simulink model "FA_18_With_Controller_Multiple_Actuator_Failure"  (R2018a)
settings: Solver=ode45  StartTime=0.0  StopTime=50  RelTol=1e-3
PreLoadFcn:
  | F18_Linear
values from neighbouring files (symbols this model uses):
  C1 = [0 -1 0 1]    [F18_Linear.m]
  d2r = pi/180    (= 0.0174532925199)    [F18_Linear.m]    (also in FA_18_Trim.m; FA_18_sfun.m; Sim.m)
  F1 = [-67.81 11973 -133.3 -11801]    [F18_Linear.m]
  F2 = 1414.2    [F18_Linear.m]
  Trimx_N = [365.74;15*d2r;0;15*d2r]    [F18_Linear.m]
undefined symbols (not defined in the file or in its folder): Earth, WGS84
libraries: aerolibfltsims x1, aerolibtransform2 x1, aerolibconvert2 x1
settings Model: Creator=User  LastModifiedBy=User

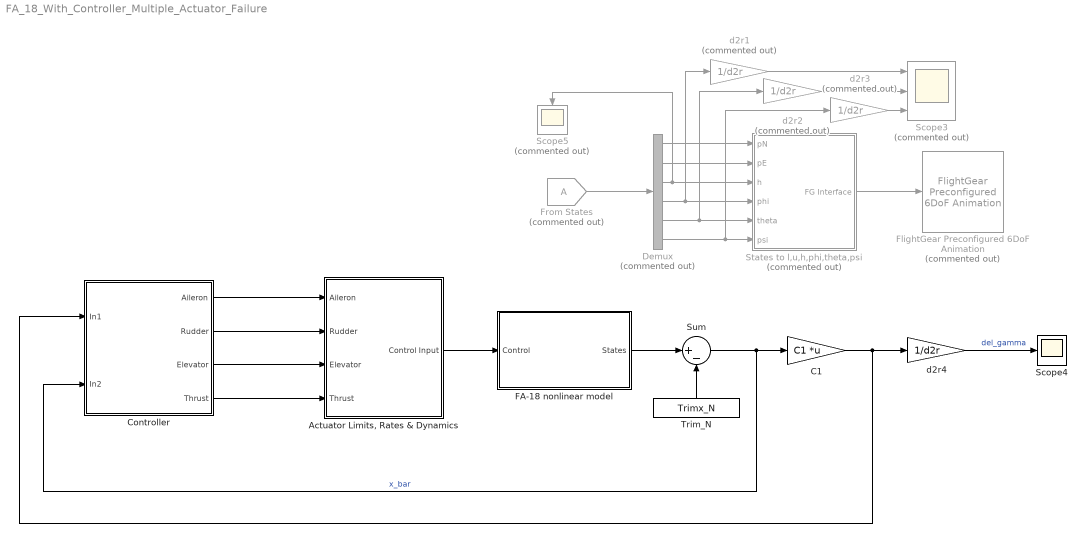
== system FA_18_With_Controller_Multiple_Actuator_Failure ==
  "Actuator Limits, Rates & Dynamics" : Subsystem
  C1 : Gain  Gain=C1  Multiplication=Matrix(K*u)
  Controller : Subsystem
  Demux : Demux  Commented=on  Outputs=6
  FA-18 nonlinear model : Subsystem
  FlightGear Preconfigured 6DoF Animation : aerolibfltsims/FlightGear Preconfigured 6DoF Animation  Commented=on  xFlightGearVersion=v2017.3  DestinationIpAddress=127.0.0.1  DestinationPort=5502  SampleTime=1/30
      settings: SourceProductName=Aerospace Blockset
  From States : From  Commented=on  TagVisibility=global
  Scope3 : Scope  Commented=on  NumInputPorts=3
  Scope4 : Scope
  Scope5 : Scope  Commented=on
  States to l,u,h,phi,theta,psi : Subsystem  Commented=on
  Sum : Sum  Inputs=|+-
  Trim_N : Constant  Value=Trimx_N
  d2r1 : Gain  Commented=on  Gain=1/d2r
  d2r2 : Gain  Commented=on  Gain=1/d2r
  d2r3 : Gain  Commented=on  Gain=1/d2r
  d2r4 : Gain  Gain=1/d2r
  wires:
  "Actuator Limits, Rates & Dynamics"/1(Control Input) -> FA-18 nonlinear model/1(Control)
  FA-18 nonlinear model/1(States) -> Sum/1
  Trim_N/1 -> Sum/2
  d2r4/1 -> Scope4/1  "del_gamma"
  C1/1 -> Controller/1(In1), d2r4/1
  Sum/1 -> Controller/2(In2), C1/1  "x_bar"
  States to l,u,h,phi,theta,psi/1(FG Interface) -> FlightGear Preconfigured 6DoF Animation/1
  From States/1 -> Demux/1
  Demux/1 -> States to l,u,h,phi,theta,psi/1(pN)
  Demux/2 -> States to l,u,h,phi,theta,psi/2(pE)
  Demux/5 -> States to l,u,h,phi,theta,psi/5(theta), d2r2/1
  Demux/6 -> d2r3/1, States to l,u,h,phi,theta,psi/6(psi)
  Demux/4 -> d2r1/1, States to l,u,h,phi,theta,psi/4(phi)
  d2r1/1 -> Scope3/1
  d2r2/1 -> Scope3/2
  d2r3/1 -> Scope3/3
  Demux/3 -> Scope5/1, States to l,u,h,phi,theta,psi/3(h)
  Controller/1(Aileron) -> "Actuator Limits, Rates & Dynamics"/1(Aileron)
  Controller/2(Rudder) -> "Actuator Limits, Rates & Dynamics"/2(Rudder)
  Controller/3("Elevator ") -> "Actuator Limits, Rates & Dynamics"/3(Elevator)
  Controller/4(Thrust) -> "Actuator Limits, Rates & Dynamics"/4(Thrust)

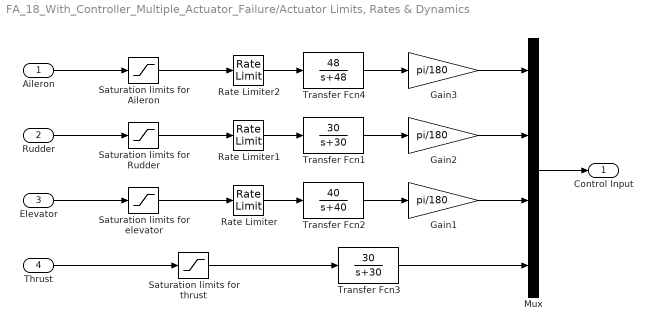
== system FA_18_With_Controller_Multiple_Actuator_Failure/Actuator Limits, Rates & Dynamics ==
  Aileron : Inport
  Rudder : Inport  Port=2
  Elevator : Inport  Port=3
  Thrust : Inport  Port=4
  Gain1 : Gain  Gain=pi/180
  Gain2 : Gain  Gain=pi/180
  Gain3 : Gain  Gain=pi/180
  Mux : Mux
  Rate Limiter : RateLimiter  RisingSlewLimit=40  FallingSlewLimit=-40  SampleTimeMode=inherited
  Rate Limiter1 : RateLimiter  RisingSlewLimit=61  FallingSlewLimit=-61  SampleTimeMode=inherited
  Rate Limiter2 : RateLimiter  RisingSlewLimit=100  FallingSlewLimit=-100  SampleTimeMode=inherited
  Saturation limits for Aileron : Saturate  UpperLimit=45  LowerLimit=-25
  Saturation limits for Rudder : Saturate  UpperLimit=30  LowerLimit=30
  Saturation limits for elevator : Saturate  UpperLimit=10.5  LowerLimit=-24
  Saturation limits for thrust : Saturate  UpperLimit=20000  LowerLimit=0
  Transfer Fcn1 : TransferFcn  Numerator=[30]  Denominator=[1 30]
  Transfer Fcn2 : TransferFcn  Numerator=[40]  Denominator=[1 40]
  Transfer Fcn3 : TransferFcn  Numerator=[30]  Denominator=[1 30]
  Transfer Fcn4 : TransferFcn  Numerator=[48]  Denominator=[1 48]
  Control Input : Outport
  wires:
  Mux/1 -> Control Input/1
  Thrust/1 -> Saturation limits for thrust/1
  Transfer Fcn3/1 -> Mux/4
  Saturation limits for thrust/1 -> Transfer Fcn3/1
  Saturation limits for elevator/1 -> Rate Limiter/1
  Rate Limiter/1 -> Transfer Fcn2/1
  Elevator/1 -> Saturation limits for elevator/1
  Gain1/1 -> Mux/3
  Transfer Fcn2/1 -> Gain1/1
  Saturation limits for Aileron/1 -> Rate Limiter2/1
  Aileron/1 -> Saturation limits for Aileron/1
  Rudder/1 -> Saturation limits for Rudder/1
  Saturation limits for Rudder/1 -> Rate Limiter1/1
  Rate Limiter1/1 -> Transfer Fcn1/1
  Rate Limiter2/1 -> Transfer Fcn4/1
  Transfer Fcn4/1 -> Gain3/1
  Transfer Fcn1/1 -> Gain2/1
  Gain2/1 -> Mux/2
  Gain3/1 -> Mux/1

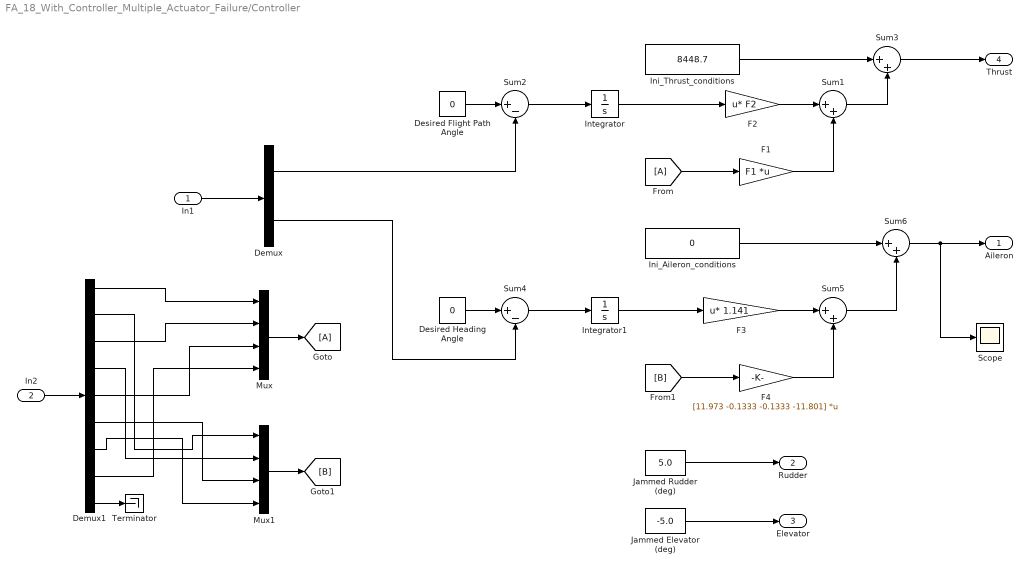
== system FA_18_With_Controller_Multiple_Actuator_Failure/Controller ==
  In1 : Inport
  In2 : Inport  Port=2
  Demux : Demux  Outputs=2
  Demux1 : Demux  Outputs=9
  Desired Flight Path Angle : Constant  Value=0
  Desired Heading Angle : Constant  Value=0
  F1 : Gain  Gain=F1  Multiplication=Matrix(K*u)
  F2 : Gain  Gain=F2  Multiplication=Matrix(u*K)
  F3 : Gain  Gain=1.141  Multiplication=Matrix(u*K)
  F4 : Gain  Gain=[11.973 -0.1333 -0.1333 -11.801]  Multiplication=Matrix(K*u)
  Ini_Aileron_conditions : Constant  Value=0
  Ini_Thrust_conditions : Constant  Value=8448.7
  Integrator : Integrator
  Integrator1 : Integrator
  Jammed Elevator (deg) : Constant  Value=-5.0
  Jammed Rudder (deg) : Constant  Value=5.0
  Mux : Mux
  Mux1 : Mux
  Scope : Scope
  Sum{1,3,5..6} (4 alike) : Sum  Inputs=|++
  Sum2 : Sum  Inputs=|+-
  Sum4 : Sum  Inputs=|+-
  Terminator : Terminator
  Aileron : Outport
  Rudder : Outport  Port=2
  "Elevator " : Outport  Port=3
  Thrust : Outport  Port=4
  wires:
  F2/1 -> Sum1/1
  Ini_Thrust_conditions/1 -> Sum3/1
  Integrator/1 -> F2/1
  Desired Flight Path Angle/1 -> Sum2/1
  Sum2/1 -> Integrator/1
  Sum1/1 -> Sum3/2
  F1/1 -> Sum1/2
  Sum3/1 -> Thrust/1
  Jammed Elevator (deg)/1 -> "Elevator "/1
  Jammed Rudder (deg)/1 -> Rudder/1
  In1/1 -> Demux/1
  Demux/1 -> Sum2/2
  Desired Heading Angle/1 -> Sum4/1
  Demux/2 -> Sum4/2
  Sum4/1 -> Integrator1/1
  Integrator1/1 -> F3/1
  F3/1 -> Sum5/1
  Sum6/1 -> Scope/1, Aileron/1
  Ini_Aileron_conditions/1 -> Sum6/1
  Sum5/1 -> Sum6/2
  F4/1 -> Sum5/2
  In2/1 -> Demux1/1
  Demux1/1 -> Mux/1
  Demux1/3 -> Mux/2
  Demux1/5 -> Mux/3
  Demux1/8 -> Mux/4
  Demux1/2 -> Mux1/1
  Demux1/4 -> Mux1/2
  Demux1/6 -> Mux1/3
  Demux1/7 -> Mux1/4
  Mux/1 -> [A]
  [A] -> F1/1
  Mux1/1 -> [B]
  [B] -> F4/1
  Demux1/9 -> Terminator/1

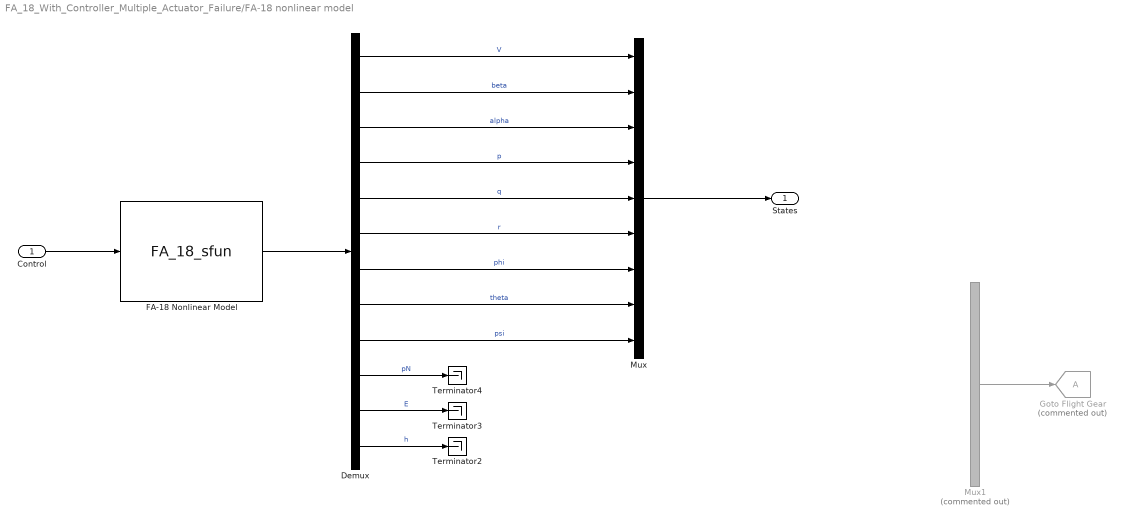
== system FA_18_With_Controller_Multiple_Actuator_Failure/FA-18 nonlinear model ==
  Control : Inport
  Demux : Demux  Outputs=12
  FA-18 Nonlinear Model : S-Function  FunctionName=FA_18_sfun  SFunctionDeploymentMode=off  EnableBusSupport=off
  Goto Flight Gear : Goto  Commented=on  TagVisibility=global
  Mux : Mux  Inputs=9
  Mux1 : Mux  Commented=on  Inputs=6
  Terminator2 : Terminator
  Terminator3 : Terminator
  Terminator4 : Terminator
  States : Outport
  wires:
  Control/1 -> FA-18 Nonlinear Model/1
  FA-18 Nonlinear Model/1 -> Demux/1
  Demux/2 -> Mux/2  "beta"
  Mux/1 -> States/1
  Demux/4 -> Mux/4  "p"
  Mux1/1 -> Goto Flight Gear/1
  Demux/1 -> Mux/1  "V"
  Demux/10 -> Terminator4/1  "pN"
  Demux/11 -> Terminator3/1  "E"
  Demux/12 -> Terminator2/1  "h"
  Demux/3 -> Mux/3  "alpha"
  Demux/5 -> Mux/5  "q"
  Demux/6 -> Mux/6  "r"
  Demux/7 -> Mux/7  "phi"
  Demux/8 -> Mux/8  "theta"
  Demux/9 -> Mux/9  "psi"

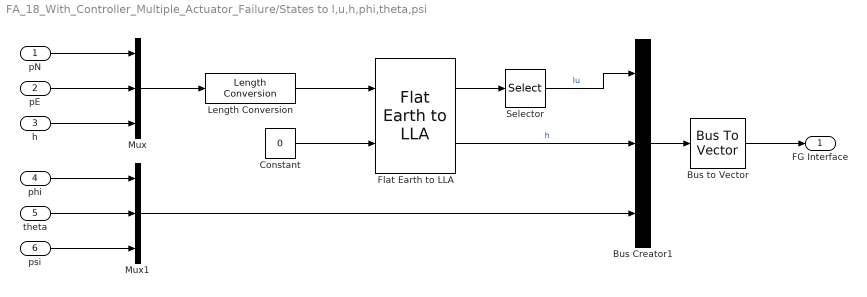
== system FA_18_With_Controller_Multiple_Actuator_Failure/States to l,u,h,phi,theta,psi ==
  pN : Inport
  pE : Inport  Port=2
  h : Inport  Port=3
  phi : Inport  Port=4
  theta : Inport  Port=5
  psi : Inport  Port=6
  Bus Creator1 : BusCreator  Inputs=3
  Bus to Vector : BusToVector
  Constant : Constant  Value=0
  Flat Earth to LLA : aerolibtransform2/Flat Earth to LLA  units=Metric (MKS)  ptype=Earth (WGS84)  F=1/298.257223563  R=6378137  LL0=[50.1018 14.2632]  psi=0
  Length Conversion : aerolibconvert2/Length Conversion  IU=ft  OU=m
  Mux : Mux  Inputs=3
  Mux1 : Mux  Inputs=3
  Selector : Selector  IndexMode=Zero-based  InputPortWidth=2  IndexOptions=Index vector (dialog)  Indices=[1 0]  OutputSizes=1
  FG Interface : Outport
  wires:
  Constant/1 -> Flat Earth to LLA/2
  Length Conversion/1 -> Flat Earth to LLA/1
  Bus to Vector/1 -> FG Interface/1
  Bus Creator1/1 -> Bus to Vector/1
  Flat Earth to LLA/1 -> Selector/1
  Selector/1 -> Bus Creator1/1  "lu"
  Flat Earth to LLA/2 -> Bus Creator1/2  "h"
  pN/1 -> Mux/1
  pE/1 -> Mux/2
  h/1 -> Mux/3
  Mux/1 -> Length Conversion/1
  theta/1 -> Mux1/2
  phi/1 -> Mux1/1
  psi/1 -> Mux1/3
  Mux1/1 -> Bus Creator1/3
